simulink model "Joystick_SIM"  (R2025b)
settings: Solver=FixedStepDiscrete  StartTime=0.0  StopTime=inf  RelTol=1e-3
undefined symbols (not defined in the file): const_voltage, sim_joy_input
settings Model: Creator=vulcangrip  LastModifiedBy=kjhaydon
settings OptimizationCC: DefaultParameterBehavior=Inlined  EnhancedBackFolding=on  PassReuseOutputArgsAs=Individual arguments  ZeroExternalMemoryAtStartup=off  ZeroInternalMemoryAtStartup=off  OptimizeBlockOrder=speed  DifferentSizesBufferReuse=on  OptimizationCustomize=off  EfficientTunableParamExpr=on
settings DebuggingCC: ParameterTunabilityLossMsg=error
settings SFSimCC: MATLABDynamicMemAlloc=off  SimTargetLang=C++  SimDLTargetLibrary=mkl-dnn
settings RTWCC: SystemTargetFile=ert.tlc  GenCodeOnly=on  TemplateMakefile=ert_default_tmf  Toolchain=CMake  TargetLang=C++  Description=Embedded Coder
settings CodeAppCC: ForceParamTrailComments=on  IgnoreCustomStorageClasses=off  OperatorAnnotations=on  SimulinkDataObjDesc=on  SFDataObjDesc=on  InsertBlockDesc=on
settings ERTTargetCC: RootIOFormat=Structure reference  ERTCustomFileTemplate=example_file_process.tlc  TargetLangStandard=C++11 (ISO)  GenerateSampleERTMain=on  CodeInterfacePackaging=C++ class  SubcomponentCodeInterfacePackaging=C++ class
settings ConfigComp: CovScope=ReferencedModels

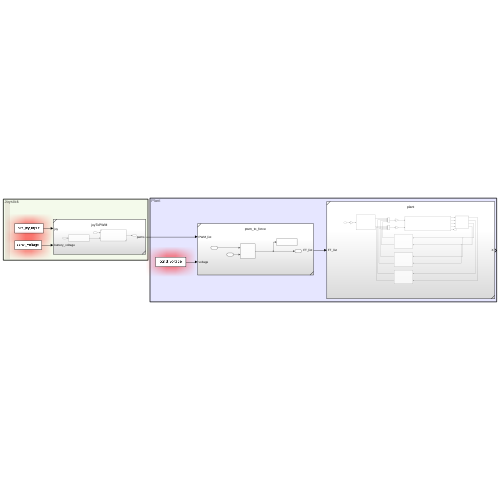
[thumbnail: Simulink's stored preview of the top-level diagram]
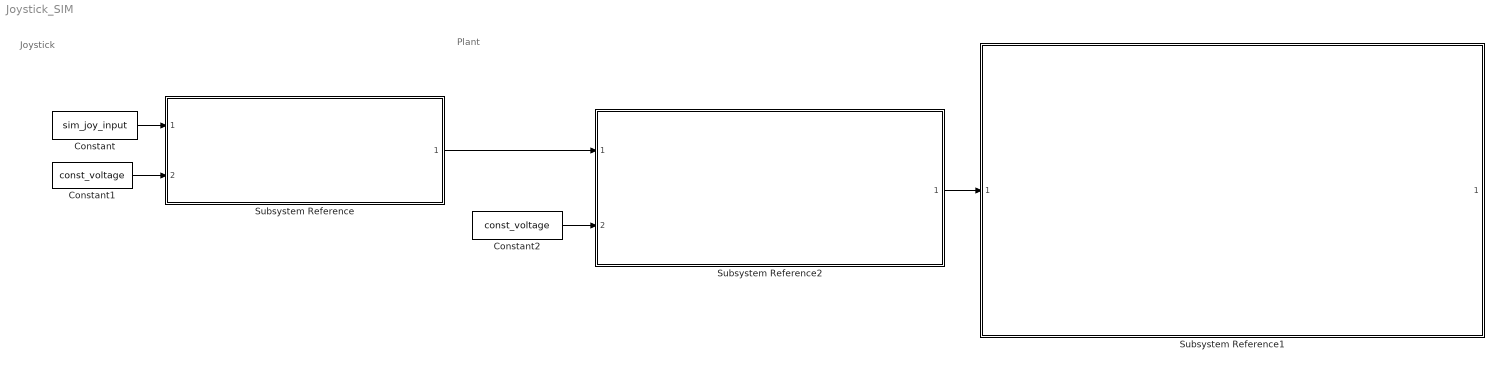
== system Joystick_SIM ==
  note: Joystick
  note: Plant
  Constant : Constant  Value=sim_joy_input
  Constant1 : Constant  Value=const_voltage
  Constant2 : Constant  Value=const_voltage
  Subsystem Reference : Subsystem  ReferencedSubsystem=joyToPWM
  Subsystem Reference1 : Subsystem  ReferencedSubsystem=plant
  Subsystem Reference2 : Subsystem  ReferencedSubsystem=pwm_to_force
  wires:
  Subsystem Reference/1 -> Subsystem Reference2/1
  Constant/1 -> Subsystem Reference/1
  Constant1/1 -> Subsystem Reference/2
  Constant2/1 -> Subsystem Reference2/2
  Subsystem Reference2/1 -> Subsystem Reference1/1
